simulink model "tank_control"  (R2019a)
settings: Solver=VariableStepAuto  StartTime=0.0  StopTime=5  RelTol=1e-3
libraries: simulink x2, simulink_extras x1
settings Model: Creator=lucas  LastModifiedBy=lucas
settings SolverCC: ZeroCrossControl=EnableAll

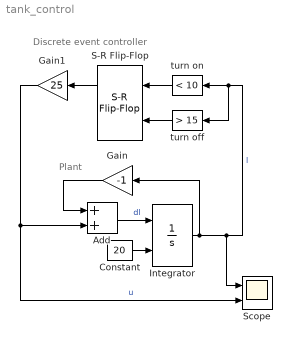
== system tank_control ==
  note: Discrete event controller
  note: Plant
  Add : Sum
  Constant : Constant  Value=20
  Gain : Gain  Gain=-1
  Gain1 : Gain  Gain=25
  Integrator : Integrator  InitialConditionSource=external  ZeroCross=off
  S-R Flip-Flop : simulink_extras/Flip Flops/S-R Flip-Flop  initial_condition=0
  Scope : Scope  NumInputPorts=2
  turn off : simulink/Logic and Bit Operations/Compare To Constant  relop=>  const=15  OutDataTypeStr=boolean
  turn on : simulink/Logic and Bit Operations/Compare To Constant  relop=<  const=10  OutDataTypeStr=boolean
  wires:
  Add/1 -> Integrator/1  "dl"
  Integrator/1 -> Scope/1, turn off/1, turn on/1, Gain/1  "l"
  Gain/1 -> Add/1
  Constant/1 -> Integrator/2
  turn off/1 -> S-R Flip-Flop/2
  turn on/1 -> S-R Flip-Flop/1
  S-R Flip-Flop/1 -> Gain1/1
  Gain1/1 -> Scope/2, Add/2  "u"
